simulink model "Quad_SF"  (Simulink 7.7)
settings: Solver=ode3  StartTime=0.0  StopTime=10.0  FixedStep=0.1  RelTol=1e-3
undefined symbols (not defined in the file or in its folder): DeltaT, H0, Kl
settings Model: Creator=Zhao Weihua  LastModifiedBy=zhao weihua

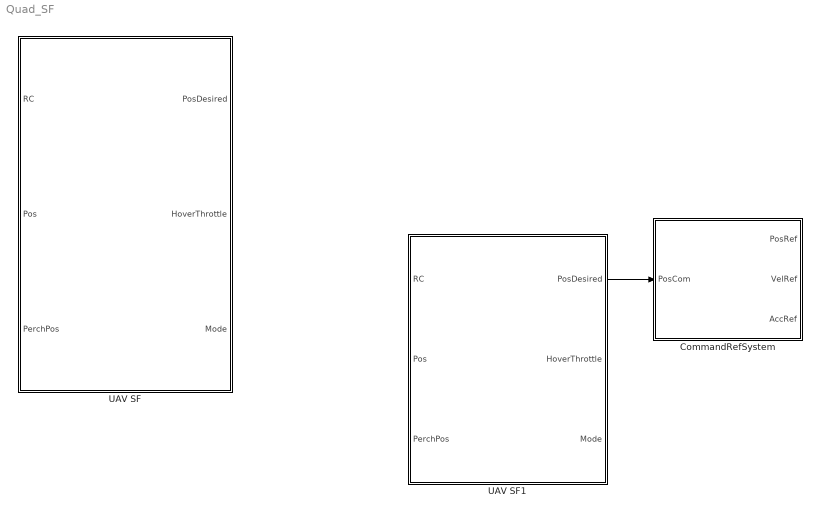
== system Quad_SF ==
  CommandRefSystem : Subsystem
  UAV SF : Stateflow chart  TreatAsAtomicUnit=on
  UAV SF1 : Stateflow chart  TreatAsAtomicUnit=on
  wires:
  UAV SF1/1(PosDesired) -> CommandRefSystem/1(PosCom)

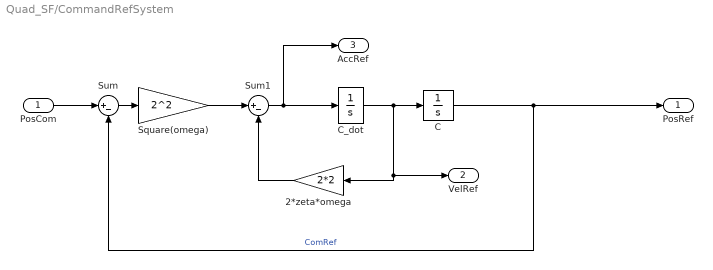
== system Quad_SF/CommandRefSystem ==
  PosCom : Inport
  2*zeta*omega : Gain  Gain=2*2
  C : Integrator
  C_dot : Integrator
  Square(omega) : Gain  Gain=2^2
  Sum : Sum  Inputs=|+-
  Sum1 : Sum  Inputs=|+-
  PosRef : Outport
  VelRef : Outport  Port=2
  AccRef : Outport  Port=3
  wires:
  C/1 -> PosRef/1, Sum/2  "ComRef"
  PosCom/1 -> Sum/1
  Sum/1 -> Square(omega)/1
  Square(omega)/1 -> Sum1/1
  C_dot/1 -> C/1, 2*zeta*omega/1, VelRef/1
  Sum1/1 -> C_dot/1, AccRef/1
  2*zeta*omega/1 -> Sum1/2

== stateflow chart UAV SF ==
  state Takeoff
    state Perching
      state Off
      state On
      On -> Off : [temp<150]
      Off -> On : [temp>=150]
      (default) -> Off
    state Trajectory
      du:
    state Hover
      du:{HoverThrottle = (H0 - HoverThrottle)*Kl*DeltaT
      + HoverThrottle ;}
    (default) -> Hover : {PosDesired = Pos;
        |   PosDesired[2] = 1;}
  state Landing
    du:{HoverThrottle = (-0.8 - HoverThrottle)*Kl*DeltaT + HoverThrottle ;}
  Landing -> Takeoff : RC[0] > 0.5
  Takeoff -> Landing : RC[0] < -0.5
  (default) -> Landing : {PosDesired = Pos;
      |   PosDesired[2] = 0; }
  data: PosDesired output double size=4; HoverThrottle output double size=1; Mode output uint8 size=3; RC input double size=5; Pos input double size=4; PerchPos input double size=4; DeltaT parameter double size=1; H0 parameter double size=1; Kl parameter double size=1

== stateflow chart UAV SF1 ==
  state In Air
    state Perching
      state Off
      state On
      On -> Off : [temp<150]
      Off -> On : [temp>=150]
      (default) -> Off
    state Trajectory
      du:
    state Take Off
      du:{HoverThrottle = (H0 - HoverThrottle)*Kl*DeltaT
      + HoverThrottle ;}
    (default) -> Take Off : {PosDesired = Pos;
        |   PosDesired[2] = 1;}
  state Landing
    du:{HoverThrottle = (-0.8 - HoverThrottle)*Kl*DeltaT + HoverThrottle ;}
  Landing -> In Air : RC[6] > 0.5
  In Air -> Landing : RC[0] < -0.5
  (default) -> Landing : {PosDesired = Pos;
      |   PosDesired[2] = 0; }
  data: PosDesired output double size=4; HoverThrottle output double size=1; Mode output uint8 size=3; RC input double size=8; Pos input double size=4; PerchPos input double size=4; DeltaT parameter double size=1; H0 parameter double size=1; Kl parameter double size=1
